simulink model "MaxonMotorModel"  (R2018a)
settings: Solver=VariableStepAuto  StartTime=0.0  StopTime=10.0  RelTol=1e-3
undefined symbols (not defined in the file or in its folder): J, Km, Kv, L, R
libraries: simulink x1
settings Model: Creator=pei-T  LastModifiedBy=pei-T

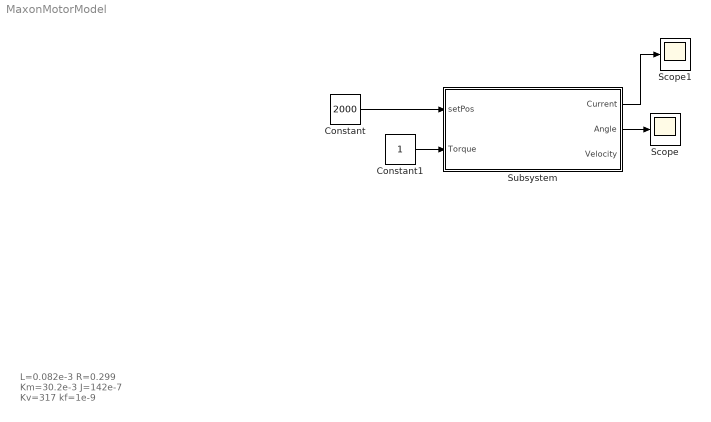
== system MaxonMotorModel ==
  note: L=0.082e-3
      | R=0.299
      | Km=30.2e-3
      | J=142e-7
      | Kv=317
      | kf=1e-9
  Constant : Constant  Value=2000
  Constant1 : Constant
  Scope : Scope
  Scope1 : Scope
  Subsystem : Subsystem
  wires:
  Constant/1 -> Subsystem/1(setPos)
  Constant1/1 -> Subsystem/2(Torque)
  Subsystem/2(Angle) -> Scope/1
  Subsystem/1(Current) -> Scope1/1

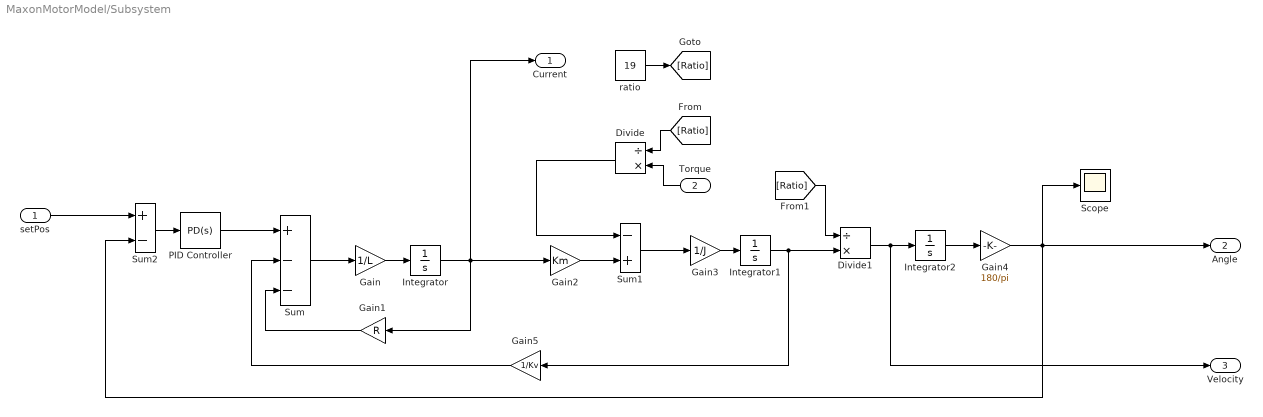
== system MaxonMotorModel/Subsystem ==
  setPos : Inport
  Torque : Inport  Port=2
  Divide : Product  Inputs=/*
  Divide1 : Product  Inputs=/*
  Gain : Gain  Gain=1/L
  Gain1 : Gain  Gain=R
  Gain2 : Gain  Gain=Km
  Gain3 : Gain  Gain=1/J
  Gain4 : Gain  Gain=180/pi
  Gain5 : Gain  Gain=1/Kv
  Integrator : Integrator  LimitOutput=on  UpperSaturationLimit=80.2  LowerSaturationLimit=-80.2
  Integrator1 : Integrator
  Integrator2 : Integrator
  PID Controller : simulink/Continuous/PID Controller  Controller=PD  TimeDomain=Continuous-time  SampleTime=-1  IntegratorMethod=Forward Euler  FilterMethod=Forward Euler  Form=Parallel  UseFilter=on  ControllerParametersSource=internal  P=0.0722255043762576  I=1  D=0.00163843606744275  N=854.573258103001  InitialConditionSource=internal  InitialConditionForIntegrator=0  InitialConditionForFilter=0  ExternalReset=none  LimitOutput=on  UpperSaturationLimit=24  LowerSaturationLimit=-24  LinearizeAsGain=on  AntiWindupMode=none  Kb=1  TrackingMode=off  Kt=1  PParamMin=[]  PParamMax=[]  IParamMin=[]  IParamMax=[]  DParamMin=[]  DParamMax=[]  NParamMin=[]  NParamMax=[]  KbParamMin=[]  KbParamMax=[]  KtParamMin=[]  KtParamMax=[]  POutMin=[]  POutMax=[]  IOutMin=[]  IOutMax=[]  DOutMin=[]  DOutMax=[]  NOutMin=[]  NOutMax=[]  KbOutMin=[]  KbOutMax=[]  KtOutMin=[]  KtOutMax=[]  IntegratorOutMin=[]  IntegratorOutMax=[]  FilterOutMin=[]  FilterOutMax=[]  SumOutMin=[]  SumOutMax=[]  SumI1OutMin=[]  SumI1OutMax=[]  SumI2OutMin=[]  SumI2OutMax=[]  SumI3OutMin=[]  SumI3OutMax=[]  SumDOutMin=[]  SumDOutMax=[]  SaturationOutMin=[]  SaturationOutMax=[]  IntegratorContinuousStateAttributes=''  IntegratorStateMustResolveToSignalObject=off  IntegratorRTWStateStorageClass=Auto  FilterContinuousStateAttributes=''  FilterStateMustResolveToSignalObject=off  FilterRTWStateStorageClass=Auto  DifferentiatorICPrevScaledInput=0  DifferentiatorOutMin=[]  DifferentiatorOutMax=[]  FilterDiffOutCoefMin=[]  FilterDiffOutCoefMax=[]  SumDenOutMin=[]  SumDenOutMax=[]  SumNumOutMin=[]  SumNumOutMax=[]  ReciprocalOutMin=[]  ReciprocalOutMax=[]  DivideOutMin=[]  DivideOutMax=[]  TunerSelectOption=Transfer Function Based (PID Tuner App)
  Scope : Scope
  Sum : Sum  Inputs=+--
  Sum1 : Sum  Inputs=-+
  Sum2 : Sum  Inputs=+-
  ratio : Constant  Value=19
  Current : Outport
  Angle : Outport  Port=2
  Velocity : Outport  Port=3
  wires:
  Integrator2/1 -> Gain4/1
  PID Controller/1 -> Sum/1
  Divide1/1 -> Velocity/1, Integrator2/1
  Gain4/1 -> Angle/1, Scope/1, Sum2/2
  Divide/1 -> Sum1/1
  [Ratio] -> Divide1/1
  Gain5/1 -> Sum/2
  Torque/1 -> Divide/2
  Gain2/1 -> Sum1/2
  setPos/1 -> Sum2/1
  Integrator/1 -> Current/1, Gain1/1, Gain2/1
  Sum2/1 -> PID Controller/1
  Integrator1/1 -> Divide1/2, Gain5/1
  Gain/1 -> Integrator/1
  Sum1/1 -> Gain3/1
  [Ratio] -> Divide/1
  Gain1/1 -> Sum/3
  Gain3/1 -> Integrator1/1
  Sum/1 -> Gain/1
  ratio/1 -> [Ratio]
